simulink model "ICARO3_orientation_controllo_BIPE"  (R2014a)
settings: Solver=FixedStepDiscrete  SolverMode=MultiTasking  StartTime=0.0  StopTime=inf  FixedStep=0.001  RelTol=1e-3
PreLoadFcn:
  | Icaro_path;
  | 
  | load_param;
  | 
  | %override compute_alloc_inside load_param !!!
  | compute_alloc_esa;
  | 
  | load('mag_calib_sim_HIL.mat');
  | 
  | init_adaptive;
InitFcn:
  | %define fast control loop sample time
  | ST = 0.005;
  | 
  | %define filters
  | s = tf('s');
  | 
  | % Derivator (useful in PID controller)
  | D = 0.01*s/(0.01*s+1);
  | 
  | % LP 2nd order filter
  | LP = 42.88/(3.5*s^2 + 19.6*s + 42.88);
  | 
  | %load new DP position controllers
  | progetto_controllo_pos_v1;
undefined symbols (not defined in the file): DiscIntNeverNeededParam, Earth, G, H, INV_PITCH_RANGE, INV_ROLL_RANGE, INV_THROTTLE_RANGE, INV_YAW_RANGE, PITCH_IDX, PITCH_MID, ROLL_IDX, ROLL_MID, RTOL, THROTTLE_DOWN, THROTTLE_IDX, THROTTLE_LOW_THRES, Ts, WGS84, YAW_IDX, YAW_MID
libraries: simulink x15, GPIO_Lib x3, cstblocks x2, aerolibtransform2 x1, STM32_Config_Lib x1
(part 5 of 5)

== system ICARO3_orientation_controllo_BIPE/SS AHRS/debias SS/Acceleration Detrend /Detrend3/Subsystem ==
  In1 : Inport
  Enable : EnablePort
  Constant : Constant
  Discrete-Time Integrator : DiscreteIntegrator  SampleTime=ST  ICPrevOutput=DiscIntNeverNeededParam  ICPrevScaledInput=DiscIntNeverNeededParam
  Discrete-Time Integrator1 : DiscreteIntegrator  InitialCondition=eps  SampleTime=ST  ICPrevOutput=DiscIntNeverNeededParam  ICPrevScaledInput=DiscIntNeverNeededParam
  Product1 : Product  Inputs=*/  SaturateOnIntegerOverflow=on  RndMeth=Zero  InputSameDT=on  OutDataTypeStr=Inherit: Same as first input
  Out2 : Outport
  wires:
  Constant/1 -> Discrete-Time Integrator1/1
  Discrete-Time Integrator1/1 -> Product1/2
  Product1/1 -> Out2/1
  Discrete-Time Integrator/1 -> Product1/1
  In1/1 -> Discrete-Time Integrator/1

== system ICARO3_orientation_controllo_BIPE/SS AHRS/debias SS/Gyros Detrend/Detrend/Subsystem ==
  In1 : Inport
  Enable : EnablePort
  Constant : Constant
  Discrete-Time Integrator : DiscreteIntegrator  SampleTime=ST  ICPrevOutput=DiscIntNeverNeededParam  ICPrevScaledInput=DiscIntNeverNeededParam
  Discrete-Time Integrator1 : DiscreteIntegrator  InitialCondition=eps  SampleTime=ST  ICPrevOutput=DiscIntNeverNeededParam  ICPrevScaledInput=DiscIntNeverNeededParam
  Product1 : Product  Inputs=*/  SaturateOnIntegerOverflow=on  RndMeth=Zero  InputSameDT=on  OutDataTypeStr=Inherit: Same as first input
  Out2 : Outport
  wires:
  In1/1 -> Discrete-Time Integrator/1
  Discrete-Time Integrator/1 -> Product1/1
  Product1/1 -> Out2/1
  Discrete-Time Integrator1/1 -> Product1/2
  Constant/1 -> Discrete-Time Integrator1/1

== system ICARO3_orientation_controllo_BIPE/SS AHRS/debias SS/Gyros Detrend/Detrend1/Subsystem ==
  In1 : Inport
  Enable : EnablePort
  Constant : Constant
  Discrete-Time Integrator : DiscreteIntegrator  SampleTime=ST  ICPrevOutput=DiscIntNeverNeededParam  ICPrevScaledInput=DiscIntNeverNeededParam
  Discrete-Time Integrator1 : DiscreteIntegrator  InitialCondition=eps  SampleTime=ST  ICPrevOutput=DiscIntNeverNeededParam  ICPrevScaledInput=DiscIntNeverNeededParam
  Product1 : Product  Inputs=*/  SaturateOnIntegerOverflow=on  RndMeth=Zero  InputSameDT=on  OutDataTypeStr=Inherit: Same as first input
  Out2 : Outport
  wires:
  Constant/1 -> Discrete-Time Integrator1/1
  Discrete-Time Integrator1/1 -> Product1/2
  Product1/1 -> Out2/1
  Discrete-Time Integrator/1 -> Product1/1
  In1/1 -> Discrete-Time Integrator/1

== system ICARO3_orientation_controllo_BIPE/SS AHRS/debias SS/Gyros Detrend/Detrend2/Subsystem ==
  In1 : Inport
  Enable : EnablePort
  Constant : Constant
  Discrete-Time Integrator : DiscreteIntegrator  SampleTime=ST  ICPrevOutput=DiscIntNeverNeededParam  ICPrevScaledInput=DiscIntNeverNeededParam
  Discrete-Time Integrator1 : DiscreteIntegrator  InitialCondition=eps  SampleTime=ST  ICPrevOutput=DiscIntNeverNeededParam  ICPrevScaledInput=DiscIntNeverNeededParam
  Product1 : Product  Inputs=*/  SaturateOnIntegerOverflow=on  RndMeth=Zero  InputSameDT=on  OutDataTypeStr=Inherit: Same as first input
  Out2 : Outport
  wires:
  In1/1 -> Discrete-Time Integrator/1
  Discrete-Time Integrator/1 -> Product1/1
  Product1/1 -> Out2/1
  Discrete-Time Integrator1/1 -> Product1/2
  Constant/1 -> Discrete-Time Integrator1/1

== matlab function ICARO3_orientation_controllo_BIPE/GPS receiver/UBLOX LEA 6 GPS/MAP ublox fix type to standard status ==
  data: u input; y output
function y = convert_gpsfix(u)
%#codegen

% Maps UBLOX gpsFix to icaro iii standard (venus gps)
% IN:
% 10 - U1 - gpsFix - GPSfix Type, range 0..5
%     0x00 = No Fix
%     0x01 = Dead Reckoning only
%     0x02 = 2D-Fix
%     0x03 = 3D-Fix
%     0x04 = GPS + dead reckoning combined
%     0x05 = Time only fix
%     0x06..0xff: reserved
% OUT: 
% 2 Fix Mode 02 Quality of fix
%     0: no fix
%     1: 2D
%     2: 3D
%     3: 3D+DGPS
%     UINT8

switch u
    case 2, y=1;
    case 3, y=2;
    otherwise y=0;
end;

== matlab function ICARO3_orientation_controllo_BIPE/sensor and actuators interface/Processing/Compensate for sensor mount _acc ==
  data: u input; y output

function y = staticAttitude(u)
%matrice rotazione
% quadrotor with DJI F450 a = 135;
% esacopter with DJI F550 a = 90;

a = 180*(pi/180);
R=[cos(a) sin(a) 0;-sin(a) cos(a) 0; 0 0 1];

y =R*u;
end

== matlab function ICARO3_orientation_controllo_BIPE/sensor and actuators interface/Processing/Compensate for sensor mount _gyro ==
  data: u input; y output
function y = staticAttitude(u)
%matrice rotazione
% quadrotor with DJI F450 a = 135;
% esacopter with DJI F550 a = 90;

a = 180*(pi/180);
R=[cos(a) sin(a) 0;-sin(a) cos(a) 0; 0 0 1];

y =R*u;
end

== matlab function ICARO3_orientation_controllo_BIPE/Compensate for sensor mount _acc1 ==
  data: u input; y output
function y = rotX(u)


R=[1 0 0;0 -1 0;0 0 -1];

y =R*u;
end

== matlab function ICARO3_orientation_controllo_BIPE/GET PPS/uint16 to vector ==
  data: gpioD input; out output
function out = fcn(gpioD)
    % assumed that gpioD is uint16
    BIT = 16;
    
    out = bitget(gpioD,1:BIT,'uint16')';

== matlab function ICARO3_orientation_controllo_BIPE/sensor and actuators interface/Processing/MATLAB Function compute magxyz2 ==
  settings: updateMethod=DISCRETE  sampleTime=ST
  data: pwms input; RC_TRPY_refs output; RC_aux_channels output; THROTTLE_IDX parameter; ROLL_IDX parameter; PITCH_IDX parameter; YAW_IDX parameter; THROTTLE_DOWN parameter; ROLL_MID parameter; PITCH_MID parameter; YAW_MID parameter; INV_THROTTLE_RANGE parameter; INV_ROLL_RANGE parameter; INV_PITCH_RANGE parameter; INV_YAW_RANGE parameter; THROTTLE_LOW_THRES parameter
function [RC_TRPY_refs,RC_aux_channels]  = compute_radio_cmds(pwms, THROTTLE_IDX, ROLL_IDX, PITCH_IDX,YAW_IDX,...
    THROTTLE_DOWN, ROLL_MID, PITCH_MID, YAW_MID,...
    INV_THROTTLE_RANGE, INV_ROLL_RANGE, INV_PITCH_RANGE, INV_YAW_RANGE,...
    THROTTLE_LOW_THRES...
)
%#codegen

%%
%%  Mange settings for different radios
%%

% RC_TRPY_refs
% 1. throttle  -> up = 1, down = 0
% 2. roll      -> left = -1, right = 1
% 3. pitch     -> up = -1, down = 1
% 4. yaw       -> left = -1, right = 1

if (1), %GENERIC RADIO WITH PARAMETRS 
    RC_TRPY_refs = [INV_THROTTLE_RANGE*(pwms(THROTTLE_IDX) - THROTTLE_DOWN);
                  INV_ROLL_RANGE*(pwms(ROLL_IDX) - ROLL_MID);
                  INV_PITCH_RANGE*(pwms(PITCH_IDX) - PITCH_MID);
                  INV_YAW_RANGE*(pwms(YAW_IDX) - YAW_MID);];


    %PATCH: this patch nulls the yaw command when the throttle
    %       is below a minimumk value in oredr to allow a safe arm, disarm
    %       procedure
    if pwms(THROTTLE_IDX) < THROTTLE_LOW_THRES,
        RC_TRPY_refs(4) = 0;
    end;
end;    


if (0), %boncioradio - Graupner MX-22 TEST JULY 2013 con radio TX-RX JETI 12 channels
    RC_TRPY_refs = [(pwms(3) - 1120)/1000;
                  -(pwms(2) - 1500)/500;
                  -(pwms(1) - 1500)/500;
                  -(pwms(4) - 1500)/500];

    %PATCH: this patch nulls the yaw command when the throttle
    %       is below a minimumk value in oredr to allow a safe arm, disarm
    %       procedure
    %NOTE: the 1130 thersold comes from the thersold used in the arm /disarm
    %detection subsystems (currently set to 1120)
    if pwms(3) < 1140,
        RC_TRPY_refs(4) = 0;
    end;
end;

if (0), %boncioradio - Graupner con radio TX-RX JETI 12 channels
    RC_TRPY_refs = [(pwms(3) - 1100)/1000;
                  -(pwms(2) - 1500)/500;
                  -(pwms(1) - 1500)/500;
                  -(pwms(4) - 1500)/500];

    %PATCH: this patch nulls the yaw command when the throttle
    %       is below a minimumk value in oredr to allow a safe arm, disarm
    %       procedure
    %NOTE: the 1130 thersold comes from the thersold used in the arm /disarm
    %detection subsystems (currently set to 1120)
    if pwms(3) < 1130,
        RC_TRPY_refs(4) = 0;
    end;
end;


if (0), %Futaba 9C con TX-RX PPM R149DP 9 channels (with THR-REV)
    RC_TRPY_refs = [(pwms(3) - 1110)/1000;
                  (pwms(1) - 1520)/500; % roll e pitch invertiti su futaba
                  (pwms(2) - 1520)/500;
                  (pwms(4) - 1520)/500];

    %PATCH: this patch nulls the yaw command when the throttle
    %       is below a minimumk value in oredr to allow a safe arm, disarm
    %       procedure
    %NOTE: the 1140 thersold comes from the thersold used in the arm /disarm
    %detection subsystems (currently set to 1120)
    if pwms(3) < 1140,
        RC_TRPY_refs(4) = 0;
    end;
end;

          
% all other channels: 1100 usec = > 0, 2100 usec => 1 
RC_aux_channels =  [(pwms(5) - 1100)/1000;
              (pwms(6) - 1100)/1000;
              (pwms(7) - 1100)/1000;
              (pwms(8) - 1100)/1000;
              (pwms(9) - 1100)/1000;
              (pwms(10) - 1100)/1000;
              (pwms(11) - 1100)/1000;
              (pwms(12) - 1100)/1000];

== matlab function ICARO3_orientation_controllo_BIPE/ generatore di riferimenti/fcn ==
  data: V_istantanea input; V_ref output; a_c input; sterzo_ref output
function [V_ref, sterzo_ref] = fcn(V_istantanea, a_c)
%#codegen
L = 0.28;
  if (V_istantanea < 1.9)%mi importa che sia circa 2 prima di iniziare l engagement così da avere angoli di sterzo non eccessivi

     V_ref = 2.1;%accelera e vai a dritto
     sterzo_ref = 0.001;
  else
     V_ref = 2.1; %una volta raggiunti i 2 m/s, mantienili e soddisfa la legge di guida usando lo sterzo
     sterzo_ref = atan((L*a_c)/((V_istantanea)^2));    
  end
end

== matlab function ICARO3_orientation_controllo_BIPE/ADIS AHRS2/Attitude Filter ADIS/DCM_MARG_QUAT/dcm_marg ==
  data: euler_out output single; a_ned output single; gyro input single; acc input single; mag input single; q input single; e_int_a input single; e_int_m input single; q_out output single; Kp parameter single; Ki parameter single; T parameter single; e_int_out_a output single; e_int_out_m output single; biases output single; e_m output
function [euler_out, a_ned, q_out, e_int_out_a, e_int_out_m, biases, e_m] = fcn(gyro, acc, mag, q, e_int_a, e_int_m, Kp, Ki, T)
%#codegen

persistent ini;

% mode == 0: magnetos' errors don't affect roll and pitch angles
% mode == 1: standard implementation, roll, pitch and yaw depend on
% acceleroters and magnetos in the same measure
mode = 0;

% Magnetos and accelerometers MUST have non null norm, if they have null
% norm an error occurred and filter probably will get confused, adjust mag
% and acc values to try to avoid filter problems. 

if (norm(acc) < 1e-4)
    acc = single([0; 0; -9.81]);
end

if (norm(mag) < 1e-4)
    %mag = single([0.234; 0.008; 0.404]);
    mag = single([0; 0.5; 0]);
    
end

% Init quaternion using the first accelerometers and magnetometers reading
% in triad algorithm.

if (isempty(ini))
    q = qtriad(acc, mag);
    ini = 1;
end

q1 = q(1);
q2 = q(2);
q3 = q(3);
q4 = q(4);


gx = gyro(1);
gy = gyro(2);
gz = gyro(3);

ax = acc(1);
ay = acc(2);
az = acc(3);

mx = mag(1);
my = mag(2);
mz = mag(3);

% Rt rotates NED to body, and obviously converts body cordinates into ned
% coordinates.
 
Rt = [1 - 2*q3^2 - 2*q4^2, 2*(q2*q3-q1*q4), 2*(q2*q4+q1*q3);
     2*(q2*q3+q1*q4), 1 - 2*q2^2 - 2*q4^2, 2*(q3*q4-q1*q2);
     2*(q2*q4-q1*q3), 2*(q3*q4+q1*q2), 1 - 2*q2^2 - 2*q3^2];
 
% Filter implementation, see article for details
 
% h = Rt*[mx; my; mz]; % mag in body frame
h = [mx; my; mz]; % tag in Deca frame

bx = sqrt(h(1)^2+h(2)^2);
bz = abs(h(3));

norm_a = sqrt(ax^2+ay^2+az^2+eps);
e_a = cross([ax ay az]'/norm_a, Rt'*[0 0 -1]'); 
% norm_m = sqrt(mx^2+my^2+mz^2+eps);
norm_m = sqrt(mx^2+my^2+eps);
norm_b = sqrt(bx^2+bz^2+eps);
% e_m = cross([mx my mz]'/norm_m, Rt'*[bx 0 bz]'/norm_b);
e_m = -1.0*cross(Rt'*[mx my 0]'/norm_m, [1 0 0]');
% e_m = cross([mx my 0]'/norm([mx my 0]), Rt'*[0 1 0]');

if (mode == 0)
     
    e_int_out_a = e_int_a + T*[e_a(1:2); 0];
    e_int_out_m = e_int_m + T*[0; 0; e_m(3)];
    
    
%     e_int_out_a = e_int_a + T*[e_a(1); e_a(2); e_a(3)];
%     e_int_out_m = e_int_m + T*[e_m(1:2); 0];
    
   g = [gx; gy; gz] + Kp*[e_a(1:2); e_m(3)] + Ki*(e_int_out_a + e_int_out_m);

else
    
    e_int_out_a = e_int_a + T*e_a;
    e_int_out_m = e_int_m + T*e_m;
    
    g = [gx; gy; gz] + Kp*(e_a + e_m) + Ki*(e_int_out_a + e_int_out_m);
    
end

gx = g(1);
gy = g(2);
gz = g(3);

% Quaternion integration

dq1 = (-q2*gx - q3*gy - q4*gz)/2;
dq2 = (q1*gx + q3*gz - q4*gy)/2;
dq3 = (q1*gy - q2*gz + q4*gx)/2;
dq4 = (q1*gz + q2*gy - q3*gx)/2;

q1 = q1 + dq1*T;
q2 = q2 + dq2*T;
q3 = q3 + dq3*T;
q4 = q4 + dq4*T;

% Quaternion normalization

norm_q = sqrt(q1*q1 + q2*q2 + q3*q3 + q4*q4);
q1 = q1 / norm_q;
q2 = q2 / norm_q;
q3 = q3 / norm_q;
q4 = q4 / norm_q;

q_out = [q1; q2; q3; q4];

% Rt rotates NED to body, and obviously converts body cordinates into ned
% coordinates.

Rt = [1 - 2*q3^2 - 2*q4^2, 2*(q2*q3-q1*q4), 2*(q2*q4+q1*q3);
     2*(q2*q3+q1*q4), 1 - 2*q2^2 - 2*q4^2, 2*(q3*q4-q1*q2);
     2*(q2*q4-q1*q3), 2*(q3*q4+q1*q2), 1 - 2*q2^2 - 2*q3^2];

% Obtain rpy angles
 
psi = atan2(2*(q2*q3+q1*q4), 1 - 2*q3^2 - 2*q4^2);
theta = atan2(-2*(q2*q4-q1*q3), sqrt((2*(q3*q4+q1*q2))^2 + (1 - 2*q2^2 - 2*q3^2)^2));
phi = atan2(2*(q3*q4+q1*q2), 1 - 2*q2^2 - 2*q3^2);

% Compute accelerations in NED

a_ned = Rt*acc;

euler_out = [phi; theta; psi];

% Suppose that mean of integral correction is bias value

biases = -Ki*(e_int_out_a + e_int_out_m);

end

function R = rotz(a)
R = [ cos(a), -sin(a), 0; sin(a), cos(a), 0 ; 0, 0, 1];
end

function R = rotx(a)
R = [ 1, 0, 0; 0, cos(a), -sin(a); 0, sin(a), cos(a);];
end

function R = roty(a)
R = [ cos(a), 0, sin(a) ; 0, 1, 0, ; -sin(a), 0, cos(a)];
end

% Triad algorithm

function q_out = qtriad(acc, mag)

ib = acc/norm(acc);
ir = [0; 0; -1];
%mb = mag;
%mr = [0.234; 0.008; 0.404];
% modifiche per vettore tag
mb = [0; sqrt((mag(1)^2) + mag(2)^2); 0];
mr = [mag(1); mag(2); 0];
jb = cross(ib,mb);
jb = jb/norm(jb);
jr = cross(ir,mr);
jr = jr/norm(jr);
kb = cross(ib,jb);
kr = cross(ir,jr);
c = (ib*ir' + jb*jr' + kb*kr')';

q1 = 0.5*sqrt(1+c(1,1)+c(2,2)+c(3,3));
q2 = 0.25/q1*(c(3,2)-c(2,3));
q3 = 0.25/q1*(c(1,3)-c(3,1));
q4 = 0.25/q1*(c(2,1)-c(1,2));

q_out = [q1 q2 q3 q4]';
    
end

== matlab function ICARO3_orientation_controllo_BIPE/Control /VectorNorm ==
  data: u input; y output
function y = norm(u)
%#codegen
% Function that computes tha norm of an input vector 
% Args:
% u: vector
% Returns:
% y = norm of input vector u

y = norm(u);

== matlab function ICARO3_orientation_controllo_BIPE/Control /atan2 ==
  data: u input; theta output
function theta = atan2(u)
%#codegen
% Function that computes tha atan2 of an input vector 
% Args:
% u: vector with u(1) = x-component, u(2) = y-component

% Returns:
% theta = atan2 of input vector u

theta = atan2(u(2), u(1));
end

== matlab function ICARO3_orientation_controllo_BIPE/Control /steer_control/Control Manager ==
  data: distance input; go output; startstop input
function go = control_stopper(distance, startstop)
%#codegen
% Function for managing the controller action
% Args:
% distance: distance from car to the waypoint
% startstop: 0 if you want to stop the car, 1 if you want the controller
%            ON
% Returns:
% go: 0 if the car is near enough to the waypoint (distance >
%     distance_threshold) or you want to stop manually the car (startstop =
%     0).
%     1 if the car is far from the waypoint (distance > distance_threshold)
%     and startstop = 1

distance_threshold = 250; %mm BIPE
if ((distance < distance_threshold) || (startstop==0))
    go = 0;
else
    go = 1;

end

== matlab function ICARO3_orientation_controllo_BIPE/Control /throttle_control /Control Manager ==
  data: distance input; go output; startstop input
function go = control_stopper(distance, startstop)
%#codegen
% Function for managing the controller action
% Args:
% distance: distance from car to the waypoint
% startstop: 0 if you want to stop the car, 1 if you want the controller
%            ON
% Returns:
% go: 0 if the car is near enough to the waypoint (distance >
%     distance_threshold) or you want to stop manually the car (startstop =
%     0).
%     1 if the car is far from the waypoint (distance > distance_threshold)
%     and startstop = 1
distance_threshold = 250; %mm %BIPE
if ((distance < distance_threshold) || (startstop==0))
    go = 0;
else
    go = 1;

end

== matlab function ICARO3_orientation_controllo_BIPE/Control /throttle_control /MATLAB Function ==
  data: prev_des_control input; current_des_control input; control output
function control= pwm_limiter(prev_des_control, current_des_control)
%#codegen
% Function that limits the rising speed of pwm value. The control is 
% limited by a ramp with angular coefficient equal to 0.1 with different
% sign if the car accelerates or decelerates
% Args:
% prev_des_control: desired control (output of the proportional
% controller) at previous time step 
% current_des_control: desired control (output of the proportional
% controller) at current time step 

zero_speed_pwm = 1.42; % ms
max_speed_pwm = 1.2; % ms
control_freq = 100 %Hz
rise_time = 5;   % sec

delta = (-max_speed_pwm + zero_speed_pwm)/ rise_time / control_freq % value to reach the max pwm within rise_time from zero_speed_pwm

cur_prev_diff = current_des_control-prev_des_control;

if (abs(cur_prev_diff) < delta)
    control = current_des_control;
else
    control = prev_des_control + sign(cur_prev_diff)*delta;
end
end

== matlab function ICARO3_orientation_controllo_BIPE/sensor and actuators interface/Processing/Compute Temperature (T) and Altitude (H)/MATLAB Function ==
  settings: sampleTime=ST
  data: UT input single; T output single; UP input single; h output single; oss input; params input single; bmp085_enabled input
function [T, h] = compute_T_P(UT, UP, oss, params, bmp085_enabled)
%#codegen


% AC1 = single(decomp(bitshift(bytes(1), 8) + bytes(2)));
% AC2 = single(decomp(bitshift(bytes(3), 8) + bytes(4)));
% AC3 = single(decomp(bitshift(bytes(5), 8) + bytes(6)));
% 
% AC4 = single(bitshift(bytes(7), 8) + bytes(8));
% AC5 = single(bitshift(bytes(9), 8) + bytes(10));
% AC6 = single(bitshift(bytes(11), 8) + bytes(12));
% 
% B1 = single(decomp(bitshift(bytes(13), 8) + bytes(14)));
% B2 = single(decomp(bitshift(bytes(15), 8) + bytes(16)));
% 
% MB = single(decomp(bitshift(bytes(17), 8) + bytes(18)));
% MC = single(decomp(bitshift(bytes(19), 8) + bytes(20)));
% MD = single(decomp(bitshift(bytes(21), 8) + bytes(22)));
% 
% params = [AC1; AC2; AC3; AC4; AC5; AC6; B1; B2; MB; MC; MD];

AC1 = params(1);
AC2 = params(2);
AC3 = params(3);
AC4 = params(4);
AC5 = params(5);
AC6 = params(6);

B1 = params(7);
B2 = params(8);

MB = params(9);
MC = params(10);
MD = params(11);

% AC1 = 9169;
% AC2 = -1269;
% AC3 = -14477;
% AC4 = 35455;
% AC5 = 24446;
% AC6 = 18385;
%
% B1 = 5498;
% B2 = 179;
%
% MB = -32768;
% MC = -11075;
% MD = 2432;

% UT = UT_bytes(1)*256 + UT_bytes(2);
% UP = (UP_bytes(1)*256*256 + UP_bytes(2)*256 + UP_bytes(3))/(2^(8 - oss));

% Invalid data
if ((UT == 0 && UP == 0) || bmp085_enabled == 0)
    T = single(0);
    h = single(0);
else
    X1 = (UT - AC6)*AC5/(2^15);
    X2 = MC*2^11/(X1 + MD);
    B5 = X1 + X2;
    T = (B5 + 8)/(2^4);
    
    B6 = B5 - 4000;
    X1 = (B2*(B6*B6/(2^12)))/(2^11);
    X2 = AC2*B6/(2^11);
    X3 = X1 + X2;
    B3 = ((AC1*4 + X3)*(2^oss) + 2)/4;
    X1 = AC3*B6/(2^13);
    X2 = (B1*(B6*B6/(2^12)))/(2^16);
    X3 = ((X1 + X2) + 2)/(2^2);
    B4 = AC4*(X3 + 32768)/(2^15);
    B7 = (UP - B3)*50000/2^oss;
    P = (B7*2)/B4;
    X1 = (P/(2^8))*(P/(2^8));
    X1 = (X1*3038)/2^16;
    X2 = (-7357*P)/(2^16);
    P = P + (X1 + X2 + 3791)/2^4;
    h = 44330*(1 - (P/101325)^(1/5.255));
end

end

% function y = decomp(u)
% 
% u = single(u);
% 
% if (u > 32767)
%     y = single(-65536 + u);
% else
%     y = single(u);
% end
% 
% end

== matlab function ICARO3_orientation_controllo_BIPE/sensor and actuators interface/Processing/Compute Temperature (T) and Altitude (H)/MATLAB Function1 ==
  settings: sampleTime=ST
  data: UT_bytes input; UT output; UP_bytes input; UP output; oss input
function [UT, UP] = compute_UT_UP(UT_bytes, UP_bytes, oss)
%#codegen

UT = bitshift(UT_bytes(1), 8) + UT_bytes(2);
%UP = bitshift(UP_bytes(1), 8) + UP_bytes(2);
UP = bitshift(bitshift(UP_bytes(1), 16) + bitshift(UP_bytes(2), 8) + UP_bytes(3),-(8 - oss));
%UP = 0;

== matlab function ICARO3_orientation_controllo_BIPE/sensor and actuators interface/Processing/MATLAB Function ==
  data: h_raw input; h_calib output; CAL_PARAM parameter
function h_calib = fcn(h_raw, CAL_PARAM)
%#codegen

h_calib=[0 0 0]';
h_calib(1) = (h_raw(1)-CAL_PARAM(1))/CAL_PARAM(4);
h_calib(2) = ((h_raw(2)-CAL_PARAM(2))/CAL_PARAM(5) - ...
    ((h_raw(1)-CAL_PARAM(1))/CAL_PARAM(4))*sin(CAL_PARAM(7)))/(cos(CAL_PARAM(7)));
h_calib(3) = ((h_raw(3)-CAL_PARAM(3))/CAL_PARAM(6) - ...
    ((h_raw(1)-CAL_PARAM(1))/CAL_PARAM(4))*sin(CAL_PARAM(8))*cos(CAL_PARAM(9)) - ...
    (sin(CAL_PARAM(9))/cos(CAL_PARAM(7)))*((h_raw(2)-CAL_PARAM(2))/CAL_PARAM(5)- ...
    (h_raw(1)-CAL_PARAM(1))/CAL_PARAM(4))*sin(CAL_PARAM(7)))/(cos(CAL_PARAM(8))*cos(CAL_PARAM(9)));

== matlab function ICARO3_orientation_controllo_BIPE/sensor and actuators interface/Processing/MATLAB Function compute accxyz ==
  settings: updateMethod=DISCRETE  sampleTime=ST
  data: u input uint16; a output single; adxl345_enabled input
function a   = compute_ACCXYZ(u, adxl345_enabled)

if (adxl345_enabled == 0)
    u = u*0;
end

ax = decomp(bitshift(u(2), 8) + u(1))/256.0*9.81;
ay = decomp(bitshift(u(4), 8) + u(3))/256.0*9.81;
az = decomp(bitshift(u(6), 8) + u(5))/256.0*9.81;

a_adxl = [ax; ay; az];

% Convert a from adxl axes to ICARO2 axes

a = [1 0 0; 0 1 0; 0 0 1]*a_adxl;
end

function y = decomp(u)
u = single(u);

if (u > 32767)
    y = single(-65536 + u);
else
    y = single(u);
end
end

== matlab function ICARO3_orientation_controllo_BIPE/sensor and actuators interface/Processing/MATLAB Function compute accxyz1 ==
  settings: updateMethod=DISCRETE  sampleTime=ST
  data: u input uint16; a output single; mpu9150_gyroacc_enabled input; t output single; g output single
function [a,t,g]   = compute_MPU9150_GYROACC(u, mpu9150_gyroacc_enabled)

if (mpu9150_gyroacc_enabled == 0)
    u = u*0;
end

%map of MPU9150 scale factors 
%ACCELEROMETER
% Full-Scale Range 
% AFS_SEL=0 ±2 g
% AFS_SEL=1 ±4 g
% AFS_SEL=2 ±8 g
% AFS_SEL=3 ±16 g
% ADC Word Length Output in two’s complement format 16 bits
% Sensitivity Scale Factor 
% AFS_SEL=0 16,384 LSB/g
% AFS_SEL=1 8,192 LSB/g
% AFS_SEL=2 4,096 LSB/g
% AFS_SEL=3 2,048 LSB/g
%
%GYROSCOPE
% Full-Scale Range 
% FS_SEL=0 ±250 º/s
% FS_SEL=1 ±500 º/s
% FS_SEL=2 ±1000 º/s
% FS_SEL=3 ±2000 º/s
% Gyroscope ADC Word Length 16 bits
% Sensitivity Scale Factor 
% FS_SEL=0 131 LSB/(º/s)
% FS_SEL=1 65.5 LSB/(º/s)
% FS_SEL=2 32.8 LSB/(º/s)
% FS_SEL=3 16.4 LSB/(º/s)

% ax = decomp(bitshift(u(1), 8) + u(2))/16384.0*9.81; %2g
% ay = decomp(bitshift(u(3), 8) + u(4))/16384.0*9.81;
% az = decomp(bitshift(u(5), 8) + u(6))/16384.0*9.81;
ax = decomp(bitshift(u(1), 8) + u(2))/8192.0*9.81; %4g
ay = decomp(bitshift(u(3), 8) + u(4))/8192.0*9.81;
az = decomp(bitshift(u(5), 8) + u(6))/8192.0*9.81;

temp = decomp(bitshift(u(7), 8) + u(8))/1; %unknown

gx = decomp(bitshift(u(9), 8) + u(10))/131.0*pi/180; % rad/sec %131 = 250 deg/sec
gy = decomp(bitshift(u(11), 8) + u(12))/131.0*pi/180;
gz = decomp(bitshift(u(13), 8) + u(14))/131.0*pi/180;

a_mpu9150 = [ax; ay; az];
g_mpu9150 = [gx; gy; gz];


% Convert a from mpu9150 axes to ICARO2 axes
%   ipotesi di montaggio 1: test preliminari
%       pettine allineato con asse X e chip sul lato di sotto 
    %OLD CONFIGURATION
%a = [0 -1 0; 1 0 0; 0 0 1]*a_mpu9150;
%g = [0 -1 0; 1 0 0; 0 0 1]*g_mpu9150;
    %NEW CONFIGURATION (24/04/2015)
a = [1 0 0; 0 -1 0; 0 0 -1]*a_mpu9150;
g = [1 0 0; 0 -1 0; 0 0 -1]*g_mpu9150;
t=temp;


end

function y = decomp(u)
u = single(u);

if (u > 32767)
    y = single(-65536 + u);
else
    y = single(u);
end
end

== matlab function ICARO3_orientation_controllo_BIPE/sensor and actuators interface/Processing/MATLAB Function compute gyroxyz ==
  settings: updateMethod=DISCRETE  sampleTime=ST
  data: u input uint16; w output single; itg3200_enabled input
function w  = compute_GYROXYZ(u, itg3200_enabled)

if (itg3200_enabled == 0)
    u = u*0;
end


wx = decomp(bitshift(u(1), 8) + u(2))*0.061*pi/180; %rad/s
wy = decomp(bitshift(u(3), 8) + u(4))*0.061*pi/180;
wz = decomp(bitshift(u(5), 8) + u(6))*0.061*pi/180;

w_itg = [wx; wy; wz];

% Convert w from itg axes to ICARO2 axes

w = [1 0 0; 0 1 0; 0 0 1]*w_itg;

end



function y = decomp(u)
u = single(u);

if (u > 32767)
    y = single(-65536 + u);
else
    y = single(u);
end
end

== matlab function ICARO3_orientation_controllo_BIPE/sensor and actuators interface/Processing/MATLAB Function compute magxyz ==
  settings: updateMethod=DISCRETE  sampleTime=ST
  data: u input uint16; m output single; hmc5833_enabled input
function m   = compute_MAGXYZ(u, hmc5833_enabled)
%#codegen

if (hmc5833_enabled == 0)
    u = u*0;
end

%note: register order is X Z Y
%OLD
% mx = decomp(bitshift(u(1), 8) + u(2))/1090;
% my = decomp(bitshift(u(3), 8) + u(4))/1090;
% mz = decomp(bitshift(u(5), 8) + u(6))/1090;
% 
% m_hmc = [mx; my; mz];
% 
% Convert m from hmc axes to ICARO2 axes
% (nota nel nuovo file)
% m = [0 0 1; -1 0 0; 0 1 0]*m_hmc;
%NEW
mx = decomp(bitshift(u(1), 8) + u(2))/1090;
mz = decomp(bitshift(u(3), 8) + u(4))/1090;
my = decomp(bitshift(u(5), 8) + u(6))/1090;
m_hmc = [mx; my; mz];

% Convert m from HMC5883 axes to dji axis
%R_x(180)
m = [1 0 0; 0 -1 0; 0 0 -1]*m_hmc;

end

function y = decomp(u)

u = single(u);

if (u > 32767)
    y = single(-65536 + u);
else
    y = single(u);
end

end

% if (my > 32767)
%     my = 65535 - my;
% end
% 
% if (mz > 32767)
%     mz = 65535 - mz;
% end

== matlab function ICARO3_orientation_controllo_BIPE/sensor and actuators interface/Processing/compute_parameters/MATLAB Function1 ==
  data: bytes input uint16; params output single size=[11 1]
function params   = compute_parameters(bytes)
%#codegen

AC1 = decomp(bitshift(bytes(1), 8) + bytes(2));
AC2 = decomp(bitshift(bytes(3), 8) + bytes(4));
AC3 = decomp(bitshift(bytes(5), 8) + bytes(6));

AC4 = single(bitshift(bytes(7), 8) + bytes(8));
AC5 = single(bitshift(bytes(9), 8) + bytes(10));
AC6 = single(bitshift(bytes(11), 8) + bytes(12));

B1 = decomp(bitshift(bytes(13), 8) + bytes(14));
B2 = decomp(bitshift(bytes(15), 8) + bytes(16));

MB = decomp(bitshift(bytes(17), 8) + bytes(18));
MC = decomp(bitshift(bytes(19), 8) + bytes(20));
MD = decomp(bitshift(bytes(21), 8) + bytes(22));

params = [AC1; AC2; AC3; AC4; AC5; AC6; B1; B2; MB; MC; MD];

end

function y = decomp(u)

u = single(u);

if (u > 32767)
    y = single(-65536 + u);
else
    y = single(u);
end

end

== matlab function ICARO3_orientation_controllo_BIPE/sensor and actuators interface/Processing/spi_data_processing/MATLAB Function compute magxyz1 ==
  settings: updateMethod=DISCRETE  sampleTime=ST
  data: u input uint16; a output single; w output single
function [a, w]  = compute_ACC_GYRO(u)
%#codegen

% Accelerations in m/s^2

ax = decomp(u(1))*2.522*9.81/1000;
ay = decomp(u(2))*2.522*9.81/1000;
az = decomp(u(3))*2.522*9.81/1000;

% PQR in rad/s

wx = decomp(u(4))*0.07326*pi/180;
wy = decomp(u(5))*0.07326*pi/180;
wz = decomp(u(6))*0.07326*pi/180;

a_adis = [ax; ay; az];
w_adis = [wx; wy; wz];

% Convert a and w from adis axes to ICARO2 axes

a = [-1 0 0; 0 1 0; 0 0 1]*a_adis;
w = [1 0 0; 0 -1 0; 0 0 -1]*w_adis;

end

function y = decomp(u)

u = single(u);

if (u > 2^13 - 1)
    y = single(-2^14 + u);
else
    y = single(u);
end

end

== matlab function ICARO3_orientation_controllo_BIPE/sensor and actuators interface/interrupt manager/CANbus data RX/Subsystem1/MATLAB Function compute gyroxyz1 ==
  settings: updateMethod=DISCRETE  sampleTime=0.01
  data: u input uint16; y output uint16
function y   = pack2_16bit(u)

y = bitor(bitshift(u(2), 8),u(1));

end

== matlab function ICARO3_orientation_controllo_BIPE/sensor and actuators interface/interrupt manager/CANbus data RX/Subsystem1/MATLAB Function compute gyroxyz2 ==
  settings: updateMethod=DISCRETE  sampleTime=0.01
  data: u input uint16; y output uint16
function y   = pack2_16bit(u)

y = bitor(bitshift(u(2), 8),u(1));

end

== matlab function ICARO3_orientation_controllo_BIPE/sensor and actuators interface/interrupt manager/CANbus data RX/Subsystem1/MATLAB Function compute gyroxyz3 ==
  settings: updateMethod=DISCRETE  sampleTime=0.01
  data: u input uint16; y output uint16
function y   = pack2_16bit(u)

y = bitor(bitshift(u(2), 8),u(1));

end

== matlab function ICARO3_orientation_controllo_BIPE/sensor and actuators interface/interrupt manager/CANbus data RX/Subsystem1/MATLAB Function compute gyroxyz5 ==
  settings: updateMethod=DISCRETE  sampleTime=0.01
  data: u input uint16; y output uint16
function y   = pack2_16bit(u)

y = bitor(bitshift(u(2), 8),u(1));

end

== matlab function ICARO3_orientation_controllo_BIPE/sensor and actuators interface/interrupt manager/CANbus data RX/Subsystem2/MATLAB Function compute gyroxyz1 ==
  settings: updateMethod=DISCRETE  sampleTime=0.01
  data: u input uint32; y output uint32 size=1
function y   = pack2_32bit(u)

y = bitshift(u(4), 24) + bitshift(u(3), 16)+ bitshift(u(2), 8)+u(1);

== matlab function ICARO3_orientation_controllo_BIPE/sensor and actuators interface/interrupt manager/CANbus data RX/Subsystem2/MATLAB Function compute gyroxyz5 ==
  settings: updateMethod=DISCRETE  sampleTime=0.01
  data: u input uint32; y output uint32 size=1
function y   = pack2_32bit(u)

y = bitshift(u(4), 24) + bitshift(u(3), 16)+ bitshift(u(2), 8)+u(1);

== matlab function ICARO3_orientation_controllo_BIPE/SS AHRS/Attitude Filter SS/DCM_MARG_QUAT/dcm_marg ==
  data: euler_out output single; a_ned output single; gyro input single; acc input single; mag input single; q input single; e_int_a input single; e_int_m input single; q_out output single; Kp parameter single; Ki parameter single; T parameter single; e_int_out_a output single; e_int_out_m output single; biases output single
function [euler_out, a_ned, q_out, e_int_out_a, e_int_out_m, biases] = fcn(gyro, acc, mag, q, e_int_a, e_int_m, Kp, Ki, T)
%#codegen

persistent ini;

% mode == 0: magnetos' errors don't affect roll and pitch angles
% mode == 1: standard implementation, roll, pitch and yaw depend on
% acceleroters and magnetos in the same measure
mode = 0;

% Magnetos and accelerometers MUST have non null norm, if they have null
% norm an error occurred and filter probably will get confused, adjust mag
% and acc values to try to avoid filter problems. 

if (norm(acc) < 1e-4)
    acc = single([0; 0; -9.81]);
end

if (norm(mag) < 1e-4)
    mag = single([0.234; 0.008; 0.404]);
end

% Init quaternion using the first accelerometers and magnetometers reading
% in triad algorithm.

if (isempty(ini))
    q = qtriad(acc, mag);
    ini = 1;
end

q1 = q(1);
q2 = q(2);
q3 = q(3);
q4 = q(4);

gx = gyro(1);
gy = gyro(2);
gz = gyro(3);

ax = acc(1);
ay = acc(2);
az = acc(3);

mx = mag(1);
my = mag(2);
mz = mag(3);

% Rt rotates NED to body, and obviously converts body cordinates into ned
% coordinates.
 
Rt = [1 - 2*q3^2 - 2*q4^2, 2*(q2*q3-q1*q4), 2*(q2*q4+q1*q3);
     2*(q2*q3+q1*q4), 1 - 2*q2^2 - 2*q4^2, 2*(q3*q4-q1*q2);
     2*(q2*q4-q1*q3), 2*(q3*q4+q1*q2), 1 - 2*q2^2 - 2*q3^2];

% Filter implementation, see article for details
 
h = Rt*[mx; my; mz];

bx = sqrt(h(1)^2+h(2)^2);
bz = abs(h(3));

norm_a = sqrt(ax^2+ay^2+az^2+eps);
e_a = cross([ax ay az]'/norm_a, Rt'*[0 0 -1]');
norm_m = sqrt(mx^2+my^2+mz^2+eps);
norm_b = sqrt(bx^2+bz^2+eps);
e_m = cross([mx my mz]'/norm_m, Rt'*[bx 0 bz]'/norm_b);

if (mode == 0)
    
    e_int_out_a = e_int_a + T*[e_a(1:2); 0];
    e_int_out_m = e_int_m + T*[0; 0; e_m(3)];
    
    g = [gx; gy; gz] + Kp*[e_a(1:2); e_m(3)] + Ki*(e_int_out_a + e_int_out_m);

else
    
    e_int_out_a = e_int_a + T*e_a;
    e_int_out_m = e_int_m + T*e_m;
    
    g = [gx; gy; gz] + Kp*(e_a + e_m) + Ki*(e_int_out_a + e_int_out_m);
    
end

gx = g(1);
gy = g(2);
gz = g(3);

% Quaternion integration

dq1 = (-q2*gx - q3*gy - q4*gz)/2;
dq2 = (q1*gx + q3*gz - q4*gy)/2;
dq3 = (q1*gy - q2*gz + q4*gx)/2;
dq4 = (q1*gz + q2*gy - q3*gx)/2;

q1 = q1 + dq1*T;
q2 = q2 + dq2*T;
q3 = q3 + dq3*T;
q4 = q4 + dq4*T;

% Quaternion normalization

norm_q = sqrt(q1*q1 + q2*q2 + q3*q3 + q4*q4);
q1 = q1 / norm_q;
q2 = q2 / norm_q;
q3 = q3 / norm_q;
q4 = q4 / norm_q;

q_out = [q1; q2; q3; q4];

% Rt rotates NED to body, and obviously converts body cordinates into ned
% coordinates.

Rt = [1 - 2*q3^2 - 2*q4^2, 2*(q2*q3-q1*q4), 2*(q2*q4+q1*q3);
     2*(q2*q3+q1*q4), 1 - 2*q2^2 - 2*q4^2, 2*(q3*q4-q1*q2);
     2*(q2*q4-q1*q3), 2*(q3*q4+q1*q2), 1 - 2*q2^2 - 2*q3^2];

% Obtain rpy angles
 
psi = atan2(2*(q2*q3+q1*q4), 1 - 2*q3^2 - 2*q4^2);
theta = atan2(-2*(q2*q4-q1*q3), sqrt((2*(q3*q4+q1*q2))^2 + (1 - 2*q2^2 - 2*q3^2)^2));
phi = atan2(2*(q3*q4+q1*q2), 1 - 2*q2^2 - 2*q3^2);

% Compute accelerations in NED

a_ned = Rt*acc;

euler_out = [phi; theta; psi];

% Suppose that mean of integral correction is bias value

biases = -Ki*(e_int_out_a + e_int_out_m);

end

function R = rotz(a)
R = [ cos(a), -sin(a), 0; sin(a), cos(a), 0 ; 0, 0, 1];
end

function R = rotx(a)
R = [ 1, 0, 0; 0, cos(a), -sin(a); 0, sin(a), cos(a);];
end

function R = roty(a)
R = [ cos(a), 0, sin(a) ; 0, 1, 0, ; -sin(a), 0, cos(a)];
end

% Triad algorithm

function q_out = qtriad(acc, mag)

ib = acc/norm(acc);
ir = [0; 0; -1];
mb = mag;
mr = [0.234; 0.008; 0.404];
jb = cross(ib,mb);
jb = jb/norm(jb);
jr = cross(ir,mr);
jr = jr/norm(jr);
kb = cross(ib,jb);
kr = cross(ir,jr);
c = (ib*ir' + jb*jr' + kb*kr')';

q1 = 0.5*sqrt(1+c(1,1)+c(2,2)+c(3,3));
q2 = 0.25/q1*(c(3,2)-c(2,3));
q3 = 0.25/q1*(c(1,3)-c(3,1));
q4 = 0.25/q1*(c(2,1)-c(1,2));

q_out = [q1 q2 q3 q4]';
    
end

== matlab function ICARO3_orientation_controllo_BIPE/sensor and actuators interface/interrupt manager/send motor commands via canbus/Subsystem10/MATLAB Function compute gyroxyz4 ==
  settings: updateMethod=DISCRETE  sampleTime=0.01
  data: u input uint8; y output uint8
function y = reorder(u)

y=uint8(zeros(1,8));
y(1)=u(1);
y(2)=u(2);
y(3)=u(3);
y(4)=u(4);
y(5)=u(5);
y(6)=u(6);
y(7)=u(7);
y(8)=u(8);

== matlab function ICARO3_orientation_controllo_BIPE/sensor and actuators interface/interrupt manager/send motor commands via canbus/Subsystem7/MATLAB Function compute gyroxyz5 ==
  settings: updateMethod=DISCRETE  sampleTime=0.01
  data: u input uint16; y output uint8
function y = pack2_8bit(u)

y =uint8([0,0]);
y(1) = bitand(u,255);
y(2) = bitshift(u,-8);

== matlab function ICARO3_orientation_controllo_BIPE/sensor and actuators interface/interrupt manager/send motor commands via canbus/Subsystem8/MATLAB Function compute gyroxyz3 ==
  settings: updateMethod=DISCRETE  sampleTime=0.01
  data: u input uint16; y output uint8
function y = pack2_8bit(u)

y =uint8([0,0]);
y(1) = bitand(u,255);
y(2) = bitshift(u,-8);
